simulink model "shipping"  (R2016b)
settings: Solver=VariableStepAuto  StartTime=0.0  StopTime=10.0  RelTol=1e-3
libraries: simulink x2
settings Model: Creator=charAn  LastModifiedBy=charAn

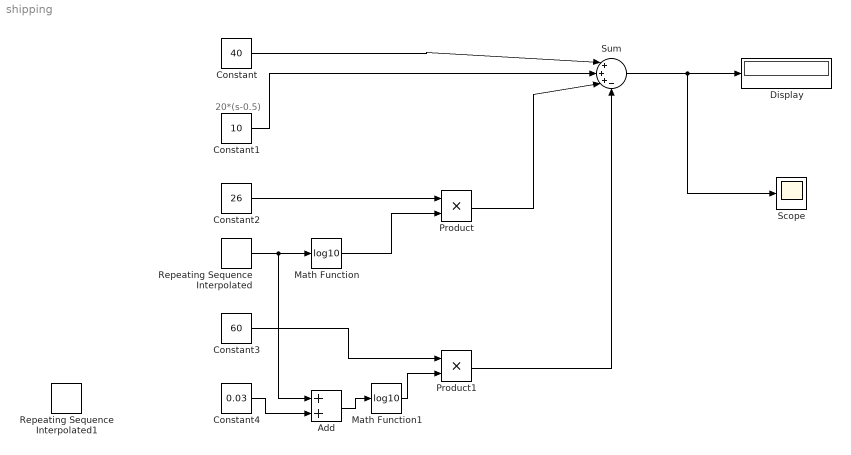
== system shipping ==
  note: 20*(s-0.5)
  Add : Sum
  Constant : Constant  Value=40
  Constant1 : Constant  Value=10
  Constant2 : Constant  Value=26
  Constant3 : Constant  Value=60
  Constant4 : Constant  Value=0.03
  Display : Display
  Math Function : Math  Operator=log10  SaturateOnIntegerOverflow=on
  Math Function1 : Math  Operator=log10  SaturateOnIntegerOverflow=on
  Product : Product
  Product1 : Product
  Repeating Sequence Interpolated : simulink/Sources/Repeating Sequence Interpolated  OutValues="[0 20 50 80 110 140 170  200]"  TimeValues=[0 10 20 30 40 50 60 70 ]  LookUpMeth=Interpolation-Use End Values  tsamp=0.01  OutMin=[]  OutMax=[]  OutDataTypeStr=double  OutputDataTypeScalingMode=double  OutDataType=fixdt(0,8)  OutScaling=2^-10
  Repeating Sequence Interpolated1 : simulink/Sources/Repeating Sequence Interpolated  OutValues="[20.03 50.03 80.03 110.03 140.03 170.03  200.03]"  TimeValues=[10 20 30 40 50 60 70]  LookUpMeth=Interpolation-Use End Values  tsamp=0.01  OutMin=[]  OutMax=[]  OutDataTypeStr=double  OutputDataTypeScalingMode=double  OutDataType=fixdt(0,8)  OutScaling=2^-10
  Scope : Scope
  Sum : Sum  Inputs=|+++-
  wires:
  Constant/1 -> Sum/1
  Constant1/1 -> Sum/2
  Product/1 -> Sum/3
  Constant2/1 -> Product/1
  Repeating Sequence Interpolated/1 -> Add/1, Math Function/1
  Math Function/1 -> Product/2
  Sum/1 -> Scope/1, Display/1
  Constant3/1 -> Product1/1
  Product1/1 -> Sum/4
  Math Function1/1 -> Product1/2
  Add/1 -> Math Function1/1
  Constant4/1 -> Add/2
